simulink model "simpleWing_example_simModel"  (R2018b)
settings: Solver=FixedStepAuto  StartTime=0.0  StopTime=10  FixedStep=0.01  RelTol=1e-3
libraries: simulink x3, axes_transformation_lib x2, flight_parameters_lib x1, simple_wing_lib x1
settings Model: Creator=Yannic  LastModifiedBy=yannic

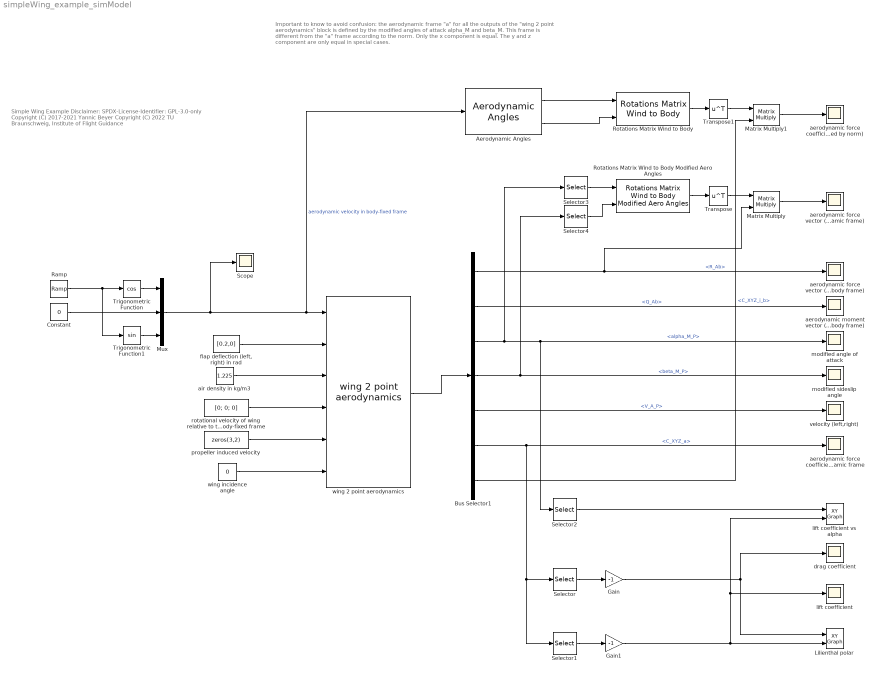
== system simpleWing_example_simModel ==
  note: Important to know to avoid confusion:
      | the aerodynamic frame "a" for all the outputs of the "wing 2 point aerodynamics" block is defined by the modified angles of attack alpha_M and beta_M.
      | This frame is different from the "a" frame according to the norm. Only the x component is equal. The y and z component are only equal in special cases.
  note: Simple Wing Example
      |
      | Disclaimer:
      | SPDX-License-Identifier: GPL-3.0-only
      |
      | Copyright (C) 2017-2021 Yannic Beyer
      | Copyright (C) 2022 TU Braunschweig, Institute of Flight Guidance
  Aerodynamic Angles : flight_parameters_lib/Aerodynamic Angles  SystemSampleTime=-1
      settings: SourceProductName=LADAC
  Bus Selector1 : BusSelector  OutputSignals=dynamicsBody.R_Ab,dynamicsBody.Q_Ab,aeroAxes.alpha_M_P,aeroAxes.beta_M_P,aeroAxes.V_A_P,dynamicsBody.C_XYZ_a,dynamicsBody.C_XYZ_i_b
  Constant : Constant  Value=0
  Gain : Gain  Gain=-1
  Gain1 : Gain  Gain=-1
  Lilienthal polar : simulink/Sinks/XY Graph  xmin=0  xmax=2  ymin=-1  ymax=1  st=-1
  Matrix Multiply : Product  Multiplication=Matrix(*)
  Matrix Multiply1 : Product  Multiplication=Matrix(*)
  Mux : Mux  Inputs=3
  Ramp : simulink/Sources/Ramp  slope=1  start=0  InitialOutput=0
  Rotations Matrix Wind to Body : axes_transformation_lib/Rotations Matrix Wind to Body  SystemSampleTime=-1
      settings: SourceProductName=LADAC
  Rotations Matrix Wind to Body Modified Aero Angles : axes_transformation_lib/Rotations Matrix Wind to Body Modified Aero Angles  SystemSampleTime=-1
      settings: SourceProductName=LADAC
  Scope : Scope
  Selector : Selector  NumberOfDimensions=2  InputPortWidth=3  IndexOptions=Index vector (dialog),Index vector (dialog)  Indices=1,1  OutputSizes=1,1
  Selector1 : Selector  NumberOfDimensions=2  InputPortWidth=3  IndexOptions=Index vector (dialog),Index vector (dialog)  Indices=3,1  OutputSizes=1,1
  Selector2 : Selector  InputPortWidth=2  IndexOptions=Index vector (dialog)  Indices=1  OutputSizes=1
  Selector3 : Selector  InputPortWidth=2  IndexOptions=Index vector (dialog)  Indices=1  OutputSizes=1
  Selector4 : Selector  InputPortWidth=2  IndexOptions=Index vector (dialog)  Indices=1  OutputSizes=1
  Transpose : Math  Operator=transpose  SaturateOnIntegerOverflow=on
  Transpose1 : Math  Operator=transpose  SaturateOnIntegerOverflow=on
  Trigonometric Function : Trigonometry  Operator=cos
  Trigonometric Function1 : Trigonometry
  aerodynamic force coefficients (as defined by norm) : Scope
  aerodynamic force coefficients in modified aerodynamic frame : Scope
  aerodynamic force vector (aerodynamic frame) : Scope
  aerodynamic force vector (body frame) : Scope
  aerodynamic moment vector (body frame) : Scope
  air density in kg/m3 : Constant  Value=1.225
  drag coefficient : Scope
  "flap deflection (left, right) in rad" : Constant  Value=[0.2,0]  VectorParams1D=off
  lift coefficient : Scope
  lift coefficient vs alpha : simulink/Sinks/XY Graph  xmin=-2  xmax=2  ymin=-1  ymax=1  st=-1
  modified angle of attack : Scope
  modified sideslip angle : Scope
  propeller induced velocity : Constant  Value=zeros(3,2)
  rotational velocity of wing relative to the air in body-fixed frame : Constant  Value=[0; 0; 0]  VectorParams1D=off
  velocity (left,right) : Scope
  wing 2 point aerodynamics : simple_wing_lib/wing 2 point aerodynamics  wing=wing  xyz_wing_c=zeros(3,1)  xyz_cg_c=zeros(3,1)
      settings: SourceProductName=LADAC
  "wing incidence angle " : Constant  Value=0
  wires:
  Mux/1 -> Scope/1, Aerodynamic Angles/1, wing 2 point aerodynamics/1  "aerodynamic velocity in body-fixed frame"
  Trigonometric Function/1 -> Mux/1
  Constant/1 -> Mux/2
  Ramp/1 -> Trigonometric Function1/1, Trigonometric Function/1
  Trigonometric Function1/1 -> Mux/3
  "flap deflection (left, right) in rad"/1 -> wing 2 point aerodynamics/2
  air density in kg/m3/1 -> wing 2 point aerodynamics/3
  rotational velocity of wing relative to the air in body-fixed frame/1 -> wing 2 point aerodynamics/4
  propeller induced velocity/1 -> wing 2 point aerodynamics/5
  "wing incidence angle "/1 -> wing 2 point aerodynamics/6
  wing 2 point aerodynamics/1 -> Bus Selector1/1
  Bus Selector1/1 -> aerodynamic force vector (body frame)/1, Matrix Multiply/2  "<R_Ab>"
  Bus Selector1/2 -> aerodynamic moment vector (body frame)/1  "<Q_Ab>"
  Bus Selector1/3 -> Selector3/1, Selector2/1, modified angle of attack/1  "<alpha_M_P>"
  Bus Selector1/5 -> velocity (left,right)/1  "<V_A_P>"
  Bus Selector1/6 -> Selector/1, Selector1/1, aerodynamic force coefficients in modified aerodynamic frame/1  "<C_XYZ_a>"
  Selector/1 -> Gain/1
  Selector1/1 -> Gain1/1
  Gain1/1 -> lift coefficient/1, lift coefficient vs alpha/2, Lilienthal polar/2
  Gain/1 -> Lilienthal polar/1, drag coefficient/1
  Selector2/1 -> lift coefficient vs alpha/1
  Rotations Matrix Wind to Body Modified Aero Angles/1 -> Transpose/1
  Transpose/1 -> Matrix Multiply/1
  Selector3/1 -> Rotations Matrix Wind to Body Modified Aero Angles/1
  Selector4/1 -> Rotations Matrix Wind to Body Modified Aero Angles/2
  Bus Selector1/4 -> modified sideslip angle/1, Selector4/1  "<beta_M_P>"
  Matrix Multiply/1 -> aerodynamic force vector (aerodynamic frame)/1
  Aerodynamic Angles/1 -> Rotations Matrix Wind to Body/1
  Aerodynamic Angles/2 -> Rotations Matrix Wind to Body/2
  Rotations Matrix Wind to Body/1 -> Transpose1/1
  Transpose1/1 -> Matrix Multiply1/1
  Bus Selector1/7 -> Matrix Multiply1/2  "<C_XYZ_i_b>"
  Matrix Multiply1/1 -> aerodynamic force coefficients (as defined by norm)/1
